simulink model "prak4"  (Simulink 7.4)
settings: Solver=ode45  StartTime=0.0  StopTime=50.0  RelTol=1e-3
libraries: vrlib x2
settings Model: Creator=Administrator  LastModifiedBy=Administrator

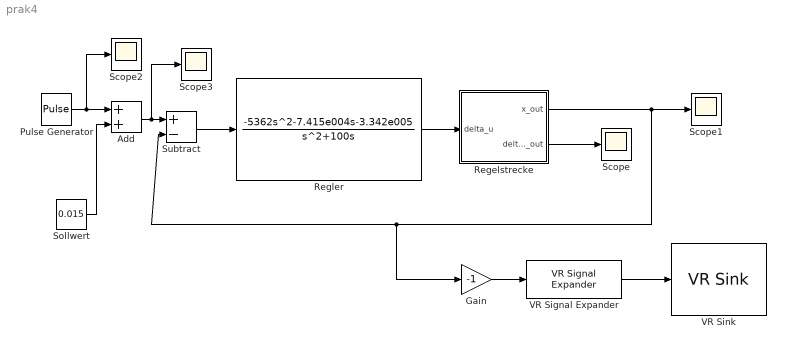
== system prak4 ==
  Add : Sum  OutDataType=fixdt(1, 16)  OutScaling=2^-10
  Gain : Gain  Gain=-1  ParameterDataType=fixdt(1, 16)  ParameterScaling=2^0  OutDataType=fixdt(1, 16)  OutScaling=2^0
  Pulse Generator : DiscretePulseGenerator  PulseType=Time based  Amplitude=0.001  Period=10  PulseWidth=50  PhaseDelay=5  SampleTime=1
  Regelstrecke : Subsystem
  Regler : TransferFcn  Numerator=[-5362 -7.415e004 -3.342e005]  Denominator=[1 100 0]
  Scope{,1..3} (4 alike) : Scope
      Scope2 settings: SaveName=ScopeData2
      Scope3 settings: SaveName=ScopeData3
  Sollwert : Constant  Value=0.015  OutDataType=fixdt(1, 16)  OutScaling=2^0
  Subtract : Sum  Inputs=+-  OutDataType=fixdt(1, 16)  OutScaling=2^-10
  VR Signal Expander : vrlib/VR Signal Expander  SystemSampleTime=-1  outwidth=3  outidx=[2]
  VR Sink : vrlib/VR Sink  InstantiateOnLoad=on  SampleTime=0.1  ViewEnable=on  RemoteChange=off  RemoteView=on  FieldsWritten=Kugel.translation.3.1.double  WorldFileName=Schwebekugel.wrl  AutoView=off  VideoDimensions=[]
  wires:
  Pulse Generator/1 -> Add/1, Scope2/1
  Regler/1 -> Regelstrecke/1(delta_u)
  Subtract/1 -> Regler/1
  Regelstrecke/1(x_out) -> Gain/1, Subtract/2, Scope1/1
  Regelstrecke/2(delta_x_out) -> Scope/1
  Gain/1 -> VR Signal Expander/1
  VR Signal Expander/1 -> VR Sink/1
  Sollwert/1 -> Add/2
  Add/1 -> Subtract/1, Scope3/1

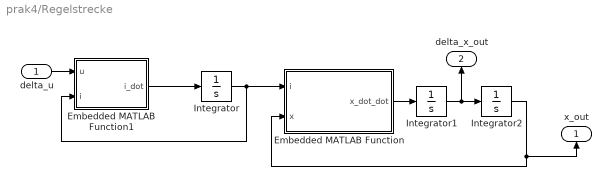
== system prak4/Regelstrecke ==
  delta_u : Inport
  Embedded MATLAB Function : Stateflow chart
  Embedded MATLAB Function1 : Stateflow chart
  Integrator : Integrator  InitialCondition=3.3221
  Integrator1 : Integrator
  Integrator2 : Integrator  InitialCondition=0.015
  x_out : Outport
  delta_x_out : Outport  Port=2
  wires:
  Embedded MATLAB Function1/1(i_dot) -> Integrator/1
  Integrator/1 -> Embedded MATLAB Function/1(i), Embedded MATLAB Function1/2(i)
  Embedded MATLAB Function/1(x_dot_dot) -> Integrator1/1
  Integrator1/1 -> Integrator2/1, delta_x_out/1
  Integrator2/1 -> Embedded MATLAB Function/2(x), x_out/1
  delta_u/1 -> Embedded MATLAB Function1/1(u)

== matlab function Regelstrecke/Embedded MATLAB Function1 ==
  data: u input double; i_dot output double; i input double
function i_dot = fcn(u, i)

R = 3;
L = 0.1;
u = u + 9.9663;

i_dot = (u - R * i) / L;

== matlab function Regelstrecke/Embedded MATLAB Function ==
  data: i input double; x_dot_dot output double; x input double
function x_dot_dot = fcn(i,x)

g = 9.81;
C = 5 * 10^-6;
m = 0.025;

x_dot_dot = g - (C * i^2)/(m * x^2);
